simulink model "PMSM_Vector_Modulation"  (R2014a)
settings: Solver=ode4  StartTime=0.0  StopTime=2  FixedStep=5e-6  RelTol=1e-3
values from neighbouring files (symbols this model uses):
  J = 0.00062    [parameter.mat]
  Ld = 0.000835    [parameter.mat]
  Lq = 0.000835    [parameter.mat]
  n_soll = 3000    [parameter.mat]
  p = 4    [parameter.mat]
  Psi_pm = 0.07147    [parameter.mat]
  R1 = 0.18    [parameter.mat]
libraries: powerlib x6, simulink x1
settings Model: Creator=benjamin  LastModifiedBy=benjamin

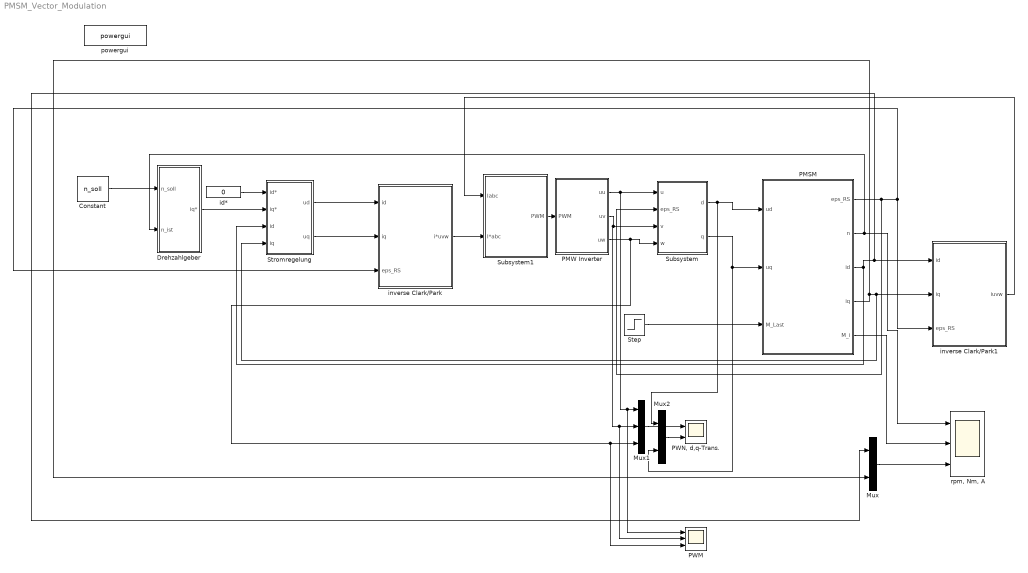
== system PMSM_Vector_Modulation ==
  Constant : Constant  Value=n_soll
  Drehzahlgeber : Subsystem
  Mux : Mux  Inputs=2
  Mux1 : Mux  Inputs=3
  Mux2 : Mux  Inputs=2
  PMSM : Subsystem
  PMW Inverter : Subsystem
  PWM : Scope  NumInputPorts=3
      settings: YMin=-100~-120~-5  YMax=100~120~5
  "PWN, d,q-Trans." : Scope  NumInputPorts=2
      settings: YMin=-100~-120  YMax=100~120
  Step : Step  After=50  SampleTime=0
  Stromregelung : Subsystem
  Subsystem : Subsystem
  Subsystem1 : Subsystem
  id* : Constant  Value=0
  inverse Clark/Park : Subsystem
  inverse Clark/Park1 : Subsystem
  powergui : powerlib/powergui  Priority=2  SimulationMode=Continuous  SolverType=Tustin  SampleTime=0  frequency=60  SPID=off  DisableSnubberDevices=off  DisableRonSwitches=off  DisableVfSwitches=off  SwTol=0  Interpol=off  DisplayEquations=off  Ts=0  methode=off  frequencyindice=0  Pbase=100e6  ErrMax=1e-4  Iterations=50  UnitsV=kV  UnitsW=MW  FunctionMessages=off  echomessages=off  HookPort=off  EnableUseOfTLC=off  x0status=blocks  RestoreLinks=warning  ResistiveCurrentMeasurement=off  Frange=logspace(0,3,50)  Ylog=off  Xlog=off  ShowGrid=off  save=off  variable=ZData  structure=0  ZoomFFT=on  StartTime=0.0  cycles=1  DisplayStyle=off  fundamental=60  FreqAxis=off  MaxFrequency=1000  frequencyindicesteady=1  RmsSteady=1  display=off
  "rpm, Nm, A" : Scope  NumInputPorts=3
      settings: TimeRange=0.1  YMin=400~22.5~-125  YMax=700~77.5~200  SaveName=ScopeData3
  wires:
  Drehzahlgeber/1(iq*) -> Stromregelung/2(iq*)
  id*/1 -> Stromregelung/1(id*)
  Stromregelung/1(ud) -> inverse Clark/Park/1(id)
  Stromregelung/2(uq) -> inverse Clark/Park/2(iq)
  PMSM/3(id) -> Mux/1, inverse Clark/Park1/1(id), Stromregelung/3(id)
  inverse Clark/Park/1(i*uvw) -> Subsystem1/2(I*abc)
  inverse Clark/Park1/1(iuvw) -> Subsystem1/1(Iabc)
  PMSM/1(eps_RS) -> Subsystem/2(eps_RS), inverse Clark/Park/3(eps_RS), inverse Clark/Park1/3(eps_RS)
  Subsystem1/1(PWM) -> PMW Inverter/1(PWM)
  PMSM/4(iq) -> Mux/2, Stromregelung/4(iq), inverse Clark/Park1/2(iq)
  PMSM/2(n) -> Drehzahlgeber/2(n_ist), "rpm, Nm, A"/1
  PMSM/5(M_i) -> "rpm, Nm, A"/2
  Mux/1 -> "rpm, Nm, A"/3
  Constant/1 -> Drehzahlgeber/1(n_soll)
  Step/1 -> PMSM/3(M_Last)
  PMW Inverter/1(uu) -> PWM/1, Mux1/1, Subsystem/1(u)
  PMW Inverter/2(uv) -> Subsystem/3(v), PWM/2, Mux1/2
  PMW Inverter/3(uw) -> PWM/3, Mux1/3, Subsystem/4(w)
  Subsystem/1(d) -> Mux2/1, PMSM/1("ud ")
  Subsystem/2(q) -> Mux2/2, PMSM/2(uq)
  Mux1/1 -> "PWN, d,q-Trans."/1
  Mux2/1 -> "PWN, d,q-Trans."/2

== system PMSM_Vector_Modulation/Drehzahlgeber ==
  n_soll : Inport
  n_ist : Inport  Port=2
  Gain : Gain  Gain=10
  Gain1 : Gain  Gain=2
  Integrator : Integrator
  Sum : Sum  Inputs=|+-
  Sum1 : Sum  Inputs=|++
  iq* : Outport
  wires:
  n_soll/1 -> Sum/1
  n_ist/1 -> Sum/2
  Sum/1 -> Gain1/1, Gain/1
  Gain/1 -> Sum1/1
  Gain1/1 -> Integrator/1
  Integrator/1 -> Sum1/2
  Sum1/1 -> iq*/1

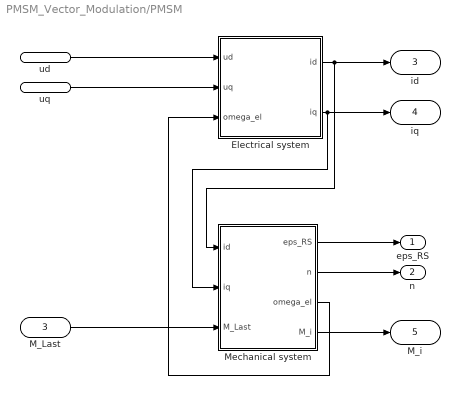
== system PMSM_Vector_Modulation/PMSM ==
  "ud " : Inport
  uq : Inport  Port=2
  M_Last : Inport  Port=3
  Electrical system : Subsystem
  Mechanical system : Subsystem
  eps_RS : Outport
  n : Outport  Port=2
  id : Outport  Port=3
  iq : Outport  Port=4
  M_i : Outport  Port=5
  wires:
  Electrical system/1(id) -> id/1, Mechanical system/1(id)
  Electrical system/2(iq) -> iq/1, Mechanical system/2(iq)
  Mechanical system/3(omega_el) -> Electrical system/3(omega_el)
  Mechanical system/1(eps_RS) -> eps_RS/1
  Mechanical system/2(n) -> n/1
  Mechanical system/4(M_i) -> M_i/1
  M_Last/1 -> Mechanical system/3(M_Last)
  uq/1 -> Electrical system/2(uq)
  "ud "/1 -> Electrical system/1(ud)

== system PMSM_Vector_Modulation/PMW Inverter ==
  PWM : Inport
  Bridge : powerlib/Power Electronics/Universal Bridge  Arms=3  SnubberResistance=1e5  SnubberCapacitance=inf  Device=MOSFET / Diodes  Ron=1e-3  Lon=0  ForwardVoltages="[  0  0  ]"  ForwardVoltage=0  GTOparameters=[ 10e-6 , 20e-6 ]  IGBTparameters=[ 1e-6 , 2e-6 ]  Measurements=None  Measurements_2=None  converterType=Rectifier
  Vdc : powerlib/Electrical Sources/DC Voltage Source  Amplitude=100  Measurements=None
  outage : Subsystem
  uu : Outport
  uv : Outport  Port=2
  uw : Outport  Port=3
  wires:
  outage/1(U12) -> uu/1
  outage/2(U23) -> uv/1
  outage/3(U31) -> uw/1
  PWM/1 -> Bridge/1
  connections:
  Bridge/LConn1 -- outage/LConn1
  Bridge/LConn2 -- outage/LConn2
  Bridge/LConn3 -- outage/LConn3
  Vdc/RConn1 -- Bridge/RConn1
  Bridge/RConn2 -- Vdc/LConn1

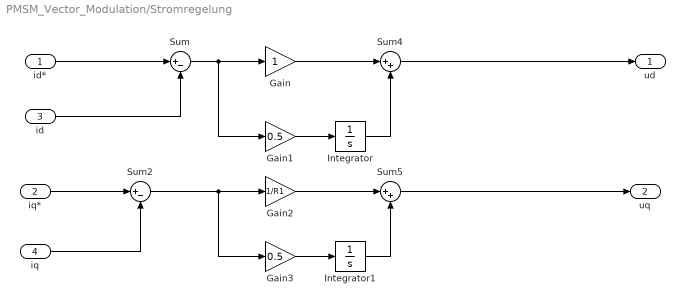
== system PMSM_Vector_Modulation/Stromregelung ==
  id* : Inport
  iq* : Inport  Port=2
  id : Inport  Port=3
  iq : Inport  Port=4
  Gain : Gain
  Gain1 : Gain  Gain=0.5
  Gain2 : Gain  Gain=1/R1
  Gain3 : Gain  Gain=0.5
  Integrator : Integrator
  Integrator1 : Integrator
  Sum : Sum  Inputs=|+-
  Sum2 : Sum  Inputs=|+-
  Sum4 : Sum  Inputs=|++
  Sum5 : Sum  Inputs=|++
  ud : Outport
  uq : Outport  Port=2
  wires:
  iq*/1 -> Sum2/1
  id*/1 -> Sum/1
  id/1 -> Sum/2
  iq/1 -> Sum2/2
  Sum/1 -> Gain1/1, Gain/1
  Gain/1 -> Sum4/1
  Gain1/1 -> Integrator/1
  Integrator/1 -> Sum4/2
  Sum2/1 -> Gain3/1, Gain2/1
  Gain2/1 -> Sum5/1
  Gain3/1 -> Integrator1/1
  Integrator1/1 -> Sum5/2
  Sum4/1 -> ud/1
  Sum5/1 -> uq/1

== system PMSM_Vector_Modulation/Subsystem ==
  u : Inport
  eps_RS : Inport  Port=2
  v : Inport  Port=3
  w : Inport  Port=4
  Clarke Transformation : Subsystem
  Park Transformation : Subsystem
  d : Outport
  q : Outport  Port=2
  wires:
  eps_RS/1 -> Park Transformation/3(epsilonRS)
  v/1 -> Clarke Transformation/2(iv)
  u/1 -> Clarke Transformation/1(iu)
  w/1 -> Clarke Transformation/3(iw)
  Clarke Transformation/2(beta) -> Park Transformation/2(beta)
  Park Transformation/1(d) -> d/1
  Park Transformation/2(q) -> q/1
  Clarke Transformation/1(alpha) -> Park Transformation/1(alpha)

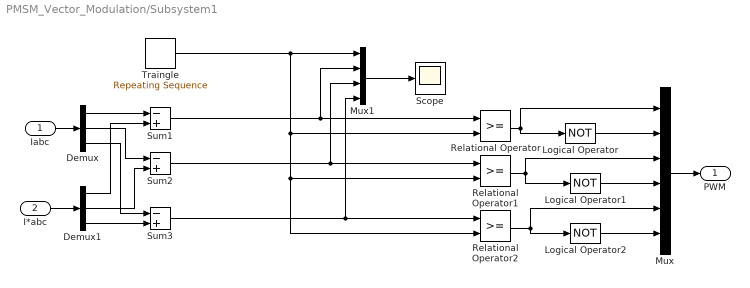
== system PMSM_Vector_Modulation/Subsystem1 ==
  Iabc : Inport
  I*abc : Inport  Port=2
  Demux : Demux  Outputs=3
  Demux1 : Demux  Outputs=3
  Logical Operator : Logic  Operator=NOT
  Logical Operator1 : Logic  Operator=NOT
  Logical Operator2 : Logic  Operator=NOT
  Mux : Mux  Inputs=6
  Mux1 : Mux
  Relational Operator : RelationalOperator  OutDataTypeStr=boolean
  Relational Operator1 : RelationalOperator  OutDataTypeStr=boolean
  Relational Operator2 : RelationalOperator  OutDataTypeStr=boolean
  Scope : Scope
      settings: YMin=-100  YMax=100  SaveName=ScopeData11
  Sum1 : Sum  Inputs=-+  SaturateOnIntegerOverflow=on  InputSameDT=on  OutDataTypeStr=Inherit: Same as first input
  Sum2 : Sum  Inputs=-+  SaturateOnIntegerOverflow=on  InputSameDT=on  OutDataTypeStr=Inherit: Same as first input
  Sum3 : Sum  Inputs=-+  SaturateOnIntegerOverflow=on  InputSameDT=on  OutDataTypeStr=Inherit: Same as first input
  Traingle : simulink/Sources/Repeating Sequence  rep_seq_t=[0 1/6000/4 3/6000/4 1/6000]  rep_seq_y=[0 -30 30 0]
  PWM : Outport
  wires:
  Iabc/1 -> Demux/1
  I*abc/1 -> Demux1/1
  Demux/1 -> Sum1/1
  Demux1/1 -> Sum1/2
  Demux/2 -> Sum2/1
  Demux1/2 -> Sum2/2
  Demux/3 -> Sum3/1
  Demux1/3 -> Sum3/2
  Relational Operator/1 -> Logical Operator/1, Mux/1
  Logical Operator/1 -> Mux/2
  Relational Operator1/1 -> Mux/3, Logical Operator1/1
  Logical Operator1/1 -> Mux/4
  Relational Operator2/1 -> Logical Operator2/1, Mux/5
  Logical Operator2/1 -> Mux/6
  Mux/1 -> PWM/1
  Sum1/1 -> Relational Operator/1, Mux1/2
  Sum2/1 -> Relational Operator1/1, Mux1/3
  Sum3/1 -> Relational Operator2/1, Mux1/4
  Traingle/1 -> Relational Operator2/2, Relational Operator1/2, Relational Operator/2, Mux1/1
  Mux1/1 -> Scope/1

== system PMSM_Vector_Modulation/inverse Clark//Park ==
  id : Inport
  iq : Inport  Port=2
  eps_RS : Inport  Port=3
  Mux : Mux  Inputs=3
  inverse Clarke Transformation : Subsystem
  inverse Park Transformation : Subsystem
  i*uvw : Outport
  wires:
  inverse Park Transformation/1(alpha) -> inverse Clarke Transformation/1(alpha)
  inverse Park Transformation/2(beta) -> inverse Clarke Transformation/2(beta)
  inverse Clarke Transformation/3(iw) -> Mux/3
  inverse Clarke Transformation/1(iu) -> Mux/1
  inverse Clarke Transformation/2(iv) -> Mux/2
  eps_RS/1 -> inverse Park Transformation/3(epsilonRS)
  id/1 -> inverse Park Transformation/1(d)
  iq/1 -> inverse Park Transformation/2(q)
  Mux/1 -> i*uvw/1

== system PMSM_Vector_Modulation/inverse Clark//Park1 ==
  id : Inport
  iq : Inport  Port=2
  eps_RS : Inport  Port=3
  Mux : Mux  Inputs=3
  inverse Clarke Transformation : Subsystem
  inverse Park Transformation : Subsystem
  iuvw : Outport
  wires:
  inverse Park Transformation/1(alpha) -> inverse Clarke Transformation/1(alpha)
  inverse Park Transformation/2(beta) -> inverse Clarke Transformation/2(beta)
  inverse Clarke Transformation/3(iw) -> Mux/3
  inverse Clarke Transformation/1(iu) -> Mux/1
  inverse Clarke Transformation/2(iv) -> Mux/2
  eps_RS/1 -> inverse Park Transformation/3(epsilonRS)
  id/1 -> inverse Park Transformation/1(d)
  iq/1 -> inverse Park Transformation/2(q)
  Mux/1 -> iuvw/1

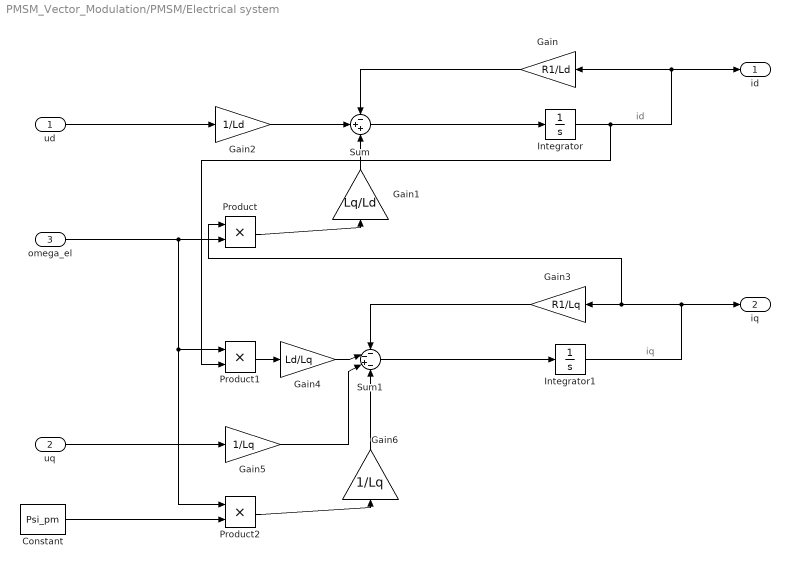
== system PMSM_Vector_Modulation/PMSM/Electrical system ==
  note: id
  note: iq
  ud : Inport
  uq : Inport  Port=2
  omega_el : Inport  Port=3
  Constant : Constant  Value=Psi_pm
  Gain : Gain  Gain=R1/Ld
  Gain1 : Gain  Gain=Lq/Ld
  Gain2 : Gain  Gain=1/Ld
  Gain3 : Gain  Gain=R1/Lq
  Gain4 : Gain  Gain=Ld/Lq
  Gain5 : Gain  Gain=1/Lq
  Gain6 : Gain  Gain=1/Lq
  Integrator : Integrator
  Integrator1 : Integrator
  Product : Product
  Product1 : Product
  Product2 : Product
  Sum : Sum  Inputs=-++
  Sum1 : Sum  Inputs=--+-
  id : Outport
  iq : Outport  Port=2
  wires:
  Sum/1 -> Integrator/1
  Integrator/1 -> Product1/2, Gain/1, id/1
  Gain/1 -> Sum/1
  omega_el/1 -> Product2/1, Product1/1, Product/2
  Gain1/1 -> Sum/3
  Product/1 -> Gain1/1
  ud/1 -> Gain2/1
  Gain2/1 -> Sum/2
  Sum1/1 -> Integrator1/1
  Integrator1/1 -> iq/1, Product/1, Gain3/1
  Gain3/1 -> Sum1/1
  Gain5/1 -> Sum1/3
  Product1/1 -> Gain4/1
  Gain4/1 -> Sum1/2
  uq/1 -> Gain5/1
  Constant/1 -> Product2/2
  Gain6/1 -> Sum1/4
  Product2/1 -> Gain6/1

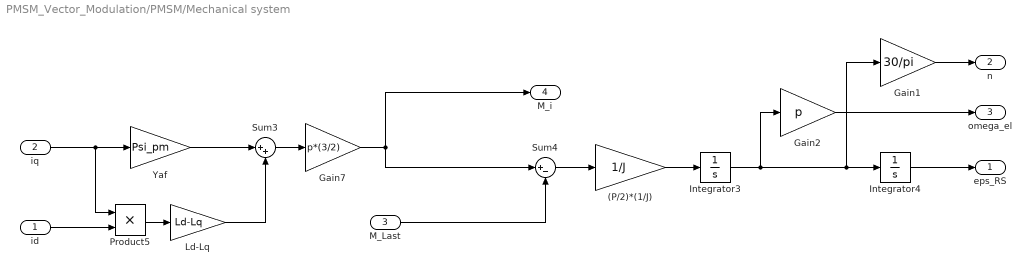
== system PMSM_Vector_Modulation/PMSM/Mechanical system ==
  id : Inport
  iq : Inport  Port=2
  M_Last : Inport  Port=3
  (P/2)*(1/J) : Gain  Gain=1/J
  Gain1 : Gain  Gain=30/pi
  Gain2 : Gain  Gain=p
  Gain7 : Gain  Gain=p*(3/2)
  Integrator3 : Integrator
  Integrator4 : Integrator
  Ld-Lq : Gain  Gain=Ld-Lq
  Product5 : Product  RndMeth=Zero
  Sum3 : Sum  Inputs=|++
  Sum4 : Sum  Inputs=|+-
  Yaf : Gain  Gain=Psi_pm
  eps_RS : Outport
  n : Outport  Port=2
  omega_el : Outport  Port=3
  M_i : Outport  Port=4
  wires:
  Yaf/1 -> Sum3/1
  Sum3/1 -> Gain7/1
  Ld-Lq/1 -> Sum3/2
  Product5/1 -> Ld-Lq/1
  Sum4/1 -> (P/2)*(1/J)/1
  iq/1 -> Product5/1, Yaf/1
  id/1 -> Product5/2
  Gain7/1 -> Sum4/1, M_i/1
  (P/2)*(1/J)/1 -> Integrator3/1
  Integrator4/1 -> eps_RS/1
  Gain1/1 -> n/1
  Integrator3/1 -> Gain1/1, Integrator4/1, Gain2/1
  M_Last/1 -> Sum4/2
  Gain2/1 -> omega_el/1

== system PMSM_Vector_Modulation/PMW Inverter/outage ==
  Voltage Measurement1 : powerlib/Measurements/Voltage Measurement  PhasorSimulation=off  OutputType=Complex  PSBequivalent=0
  Voltage Measurement2 : powerlib/Measurements/Voltage Measurement  PhasorSimulation=off  OutputType=Complex  PSBequivalent=0
  Voltage Measurement3 : powerlib/Measurements/Voltage Measurement  PhasorSimulation=off  OutputType=Complex  PSBequivalent=0
  A : PMIOPort  Port=1  Side=Left
  B : PMIOPort  Port=2  Side=Left
  C : PMIOPort  Port=3  Side=Left
  U12 : Outport
  U23 : Outport  Port=2
  U31 : Outport  Port=3
  wires:
  Voltage Measurement2/1 -> U12/1
  Voltage Measurement1/1 -> U23/1
  Voltage Measurement3/1 -> U31/1
  connections:
  Voltage Measurement1/LConn1 -- Voltage Measurement2/LConn2 -- B/RConn1
  A/RConn1 -- Voltage Measurement2/LConn1 -- Voltage Measurement3/LConn2
  C/RConn1 -- Voltage Measurement1/LConn2 -- Voltage Measurement3/LConn1

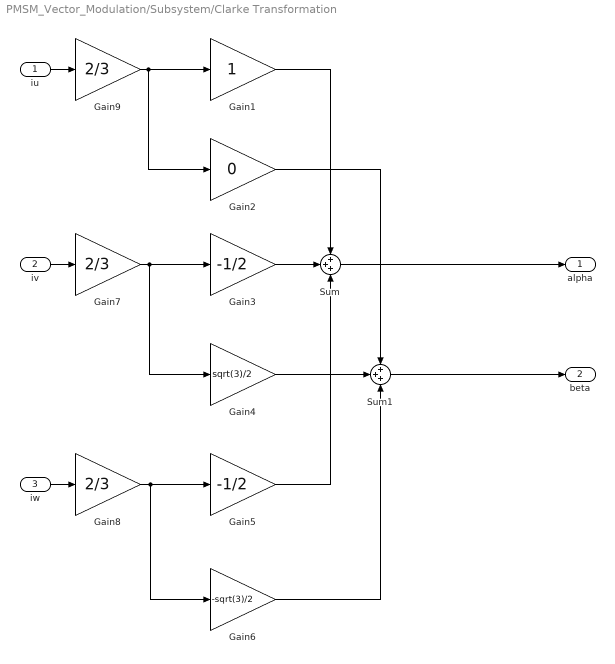
== system PMSM_Vector_Modulation/Subsystem/Clarke Transformation ==
  iu : Inport
  iv : Inport  Port=2
  iw : Inport  Port=3
  Gain1 : Gain
  "Gain2 " : Gain  Gain=0
  Gain3 : Gain  Gain=-1/2
  Gain4 : Gain  Gain=sqrt(3)/2
  Gain5 : Gain  Gain=-1/2
  Gain6 : Gain  Gain=-sqrt(3)/2
  Gain7 : Gain  Gain=2/3
  Gain8 : Gain  Gain=2/3
  Gain9 : Gain  Gain=2/3
  Sum : Sum  Inputs=+++
  Sum1 : Sum  Inputs=+++
  alpha : Outport
  beta : Outport  Port=2
  wires:
  "Gain2 "/1 -> Sum1/1
  Gain1/1 -> Sum/1
  Gain4/1 -> Sum1/2
  Gain5/1 -> Sum/3
  iw/1 -> Gain8/1
  Gain3/1 -> Sum/2
  Gain7/1 -> Gain4/1, Gain3/1
  Gain9/1 -> "Gain2 "/1, Gain1/1
  Gain8/1 -> Gain6/1, Gain5/1
  Sum/1 -> alpha/1
  Sum1/1 -> beta/1
  iv/1 -> Gain7/1
  Gain6/1 -> Sum1/3
  iu/1 -> Gain9/1

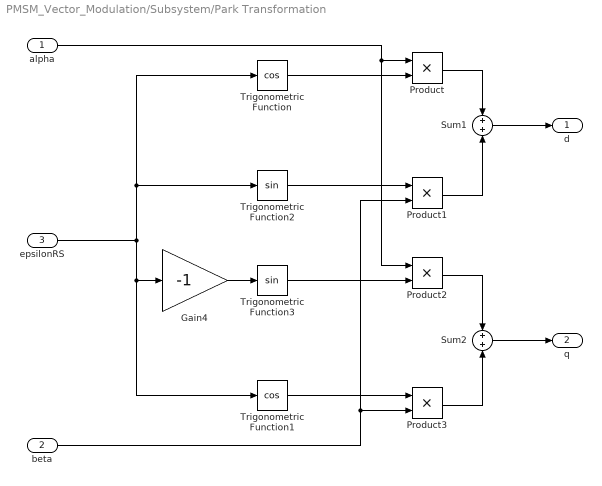
== system PMSM_Vector_Modulation/Subsystem/Park Transformation ==
  alpha : Inport
  beta : Inport  Port=2
  epsilonRS : Inport  Port=3
  Gain4 : Gain  Gain=-1
  Product{,1..3} (4 alike) : Product
  Sum1 : Sum
  Sum2 : Sum
  Trigonometric Function : Trigonometry  Operator=cos
  Trigonometric Function1 : Trigonometry  Operator=cos
  Trigonometric Function2 : Trigonometry
  Trigonometric Function3 : Trigonometry
  d : Outport
  q : Outport  Port=2
  wires:
  Sum2/1 -> q/1
  Product2/1 -> Sum2/1
  Product1/1 -> Sum1/2
  epsilonRS/1 -> Trigonometric Function2/1, Trigonometric Function/1, Gain4/1, Trigonometric Function1/1
  Trigonometric Function/1 -> Product/2
  alpha/1 -> Product2/1, Product/1
  Sum1/1 -> d/1
  Trigonometric Function1/1 -> Product3/1
  beta/1 -> Product3/2, Product1/2
  Product/1 -> Sum1/1
  Trigonometric Function2/1 -> Product1/1
  Trigonometric Function3/1 -> Product2/2
  Product3/1 -> Sum2/2
  Gain4/1 -> Trigonometric Function3/1

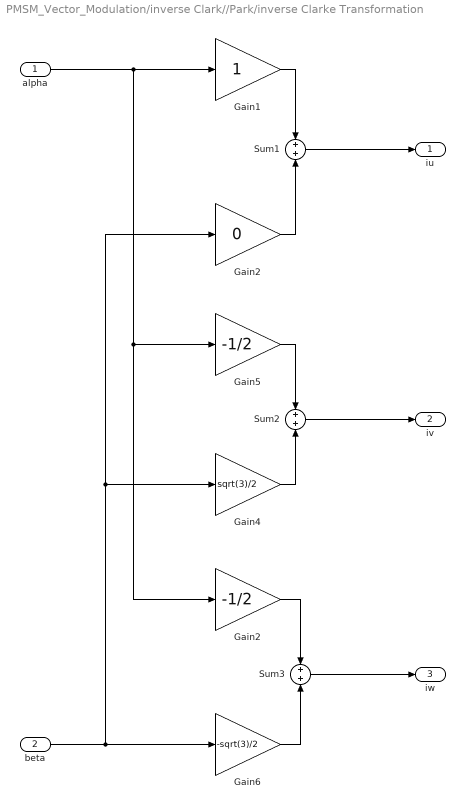
== system PMSM_Vector_Modulation/inverse Clark//Park/inverse Clarke Transformation ==
  alpha : Inport
  beta : Inport  Port=2
  Gain1 : Gain
  Gain2 : Gain  Gain=-1/2
  "Gain2 " : Gain  Gain=0
  Gain4 : Gain  Gain=sqrt(3)/2
  Gain5 : Gain  Gain=-1/2
  Gain6 : Gain  Gain=-sqrt(3)/2
  Sum1 : Sum
  Sum2 : Sum
  Sum3 : Sum
  iu : Outport
  iv : Outport  Port=2
  iw : Outport  Port=3
  wires:
  Sum2/1 -> iv/1
  beta/1 -> "Gain2 "/1, Gain4/1, Gain6/1
  Gain4/1 -> Sum2/2
  Sum1/1 -> iu/1
  "Gain2 "/1 -> Sum1/2
  Gain5/1 -> Sum2/1
  Gain1/1 -> Sum1/1
  Gain2/1 -> Sum3/1
  Gain6/1 -> Sum3/2
  alpha/1 -> Gain1/1, Gain2/1, Gain5/1
  Sum3/1 -> iw/1

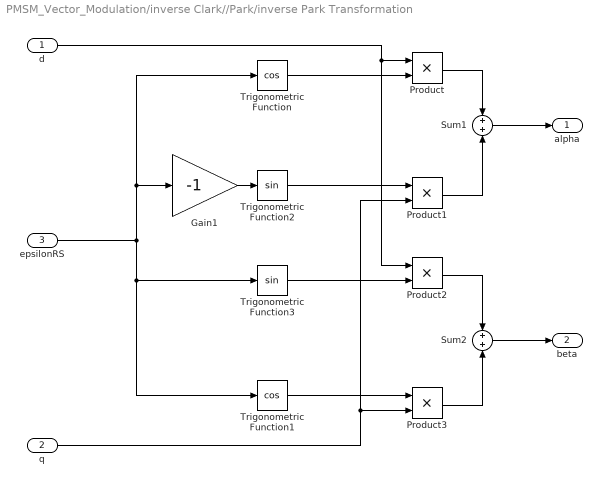
== system PMSM_Vector_Modulation/inverse Clark//Park/inverse Park Transformation ==
  d : Inport
  q : Inport  Port=2
  epsilonRS : Inport  Port=3
  Gain1 : Gain  Gain=-1
  Product{,1..3} (4 alike) : Product
  Sum1 : Sum
  Sum2 : Sum
  Trigonometric Function : Trigonometry  Operator=cos
  Trigonometric Function1 : Trigonometry  Operator=cos
  Trigonometric Function2 : Trigonometry
  Trigonometric Function3 : Trigonometry
  alpha : Outport
  beta : Outport  Port=2
  wires:
  Sum2/1 -> beta/1
  Product2/1 -> Sum2/1
  Product1/1 -> Sum1/2
  epsilonRS/1 -> Gain1/1, Trigonometric Function/1, Trigonometric Function3/1, Trigonometric Function1/1
  Trigonometric Function/1 -> Product/2
  d/1 -> Product2/1, Product/1
  Sum1/1 -> alpha/1
  Trigonometric Function1/1 -> Product3/1
  q/1 -> Product3/2, Product1/2
  Product/1 -> Sum1/1
  Trigonometric Function2/1 -> Product1/1
  Trigonometric Function3/1 -> Product2/2
  Product3/1 -> Sum2/2
  Gain1/1 -> Trigonometric Function2/1

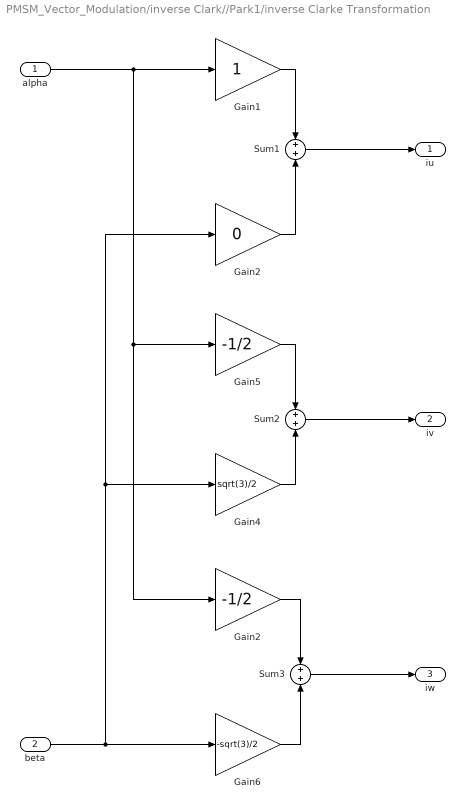
== system PMSM_Vector_Modulation/inverse Clark//Park1/inverse Clarke Transformation ==
  alpha : Inport
  beta : Inport  Port=2
  Gain1 : Gain
  Gain2 : Gain  Gain=-1/2
  "Gain2 " : Gain  Gain=0
  Gain4 : Gain  Gain=sqrt(3)/2
  Gain5 : Gain  Gain=-1/2
  Gain6 : Gain  Gain=-sqrt(3)/2
  Sum1 : Sum
  Sum2 : Sum
  Sum3 : Sum
  iu : Outport
  iv : Outport  Port=2
  iw : Outport  Port=3
  wires:
  Sum2/1 -> iv/1
  beta/1 -> "Gain2 "/1, Gain4/1, Gain6/1
  Gain4/1 -> Sum2/2
  Sum1/1 -> iu/1
  "Gain2 "/1 -> Sum1/2
  Gain5/1 -> Sum2/1
  Gain1/1 -> Sum1/1
  Gain2/1 -> Sum3/1
  Gain6/1 -> Sum3/2
  alpha/1 -> Gain1/1, Gain2/1, Gain5/1
  Sum3/1 -> iw/1

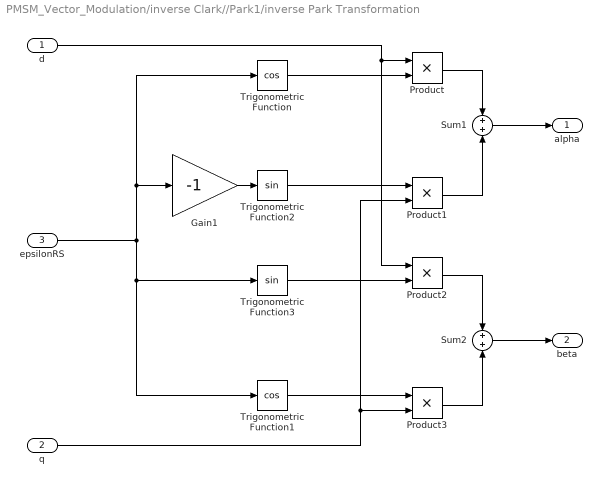
== system PMSM_Vector_Modulation/inverse Clark//Park1/inverse Park Transformation ==
  d : Inport
  q : Inport  Port=2
  epsilonRS : Inport  Port=3
  Gain1 : Gain  Gain=-1
  Product{,1..3} (4 alike) : Product
  Sum1 : Sum
  Sum2 : Sum
  Trigonometric Function : Trigonometry  Operator=cos
  Trigonometric Function1 : Trigonometry  Operator=cos
  Trigonometric Function2 : Trigonometry
  Trigonometric Function3 : Trigonometry
  alpha : Outport
  beta : Outport  Port=2
  wires:
  Sum2/1 -> beta/1
  Product2/1 -> Sum2/1
  Product1/1 -> Sum1/2
  epsilonRS/1 -> Gain1/1, Trigonometric Function/1, Trigonometric Function3/1, Trigonometric Function1/1
  Trigonometric Function/1 -> Product/2
  d/1 -> Product2/1, Product/1
  Sum1/1 -> alpha/1
  Trigonometric Function1/1 -> Product3/1
  q/1 -> Product3/2, Product1/2
  Product/1 -> Sum1/1
  Trigonometric Function2/1 -> Product1/1
  Trigonometric Function3/1 -> Product2/2
  Product3/1 -> Sum2/2
  Gain1/1 -> Trigonometric Function2/1
